simulink model "c28x_xcp_can_3pcaltool"  (R2021b)
settings: Solver=FixedStepDiscrete  StartTime=0.0  StopTime=Inf  RelTol=1e-3  EnableMultiTasking=on
model workspace (MAT data in the model file):
  COUNTER_INCR = Simulink.Parameter
  COUNTER_INCR.Value = 1
  COUNTER_INCR.DataType = 'uint16'
  COUNTER_INCR.Complexity = 'real'
  COUNTER_INCR.Dimensions = [1 1]
  STEP_PARAM = Simulink.Parameter
  STEP_PARAM.Value = 5
  STEP_PARAM.DataType = 'int16'
  STEP_PARAM.Complexity = 'real'
  STEP_PARAM.Dimensions = [1 1]
values from neighbouring files (symbols this model uses):
  STEP_PARAM = tic2000demospkg.Parameter    [c2000_ccp_data.m]
libraries: demo_controls x1
settings Model: ExtModeTrigDuration=8  Creator=The MathWorks, Inc.  LastModifiedBy=The MathWorks, Inc.
settings SolverCC: AlgebraicLoopSolver=TrustRegion  PositivePriorityOrder=on
settings OptimizationCC: DefaultParameterBehavior=Inlined  DefaultUnderspecifiedDataType=single  EnhancedBackFolding=on  PassReuseOutputArgsAs=Individual arguments  MaxStackSize=1024  OptimizeBlockOrder=speed  DifferentSizesBufferReuse=on  OptimizationCustomize=off  DenormalBehavior=FlushToZero  EfficientTunableParamExpr=on
settings DebuggingCC: ParameterTunabilityLossMsg=error  SFMachineParentedDataDiag=warning
settings HardwareCC: ProdBitPerChar=16  ProdBitPerInt=16  ProdBitPerPointer=32  ProdBitPerSizeT=32  ProdBitPerPtrDiffT=32  ProdLargestAtomicInteger=Integer  ProdLargestAtomicFloat=None  ProdWordSize=16  ProdLongLongMode=on  ProdHWDeviceType=Texas Instruments->C2000
settings SFSimCC: MATLABDynamicMemAlloc=off
settings RTWCC: Description=Embedded Coder  SystemTargetFile=ert.tlc  HardwareBoard=TI Delfino F28379D LaunchPad  TemplateMakefile=ert_default_tmf  Toolchain=Texas Instruments Code Composer Studio (C2000)
settings CodeAppCC: ForceParamTrailComments=on  IgnoreCustomStorageClasses=off  OperatorAnnotations=on  SimulinkDataObjDesc=on  SFDataObjDesc=on  InsertBlockDesc=on
settings ERTTargetCC: CodeReplacementLibrary=TI C28x  ExtModeTransport=5  ExtModeStaticAlloc=on  ExtModeStaticAllocSize=10000  ExtModeMexFile=ext_xcp  ExtModeIntrfLevel=Level2 - Open

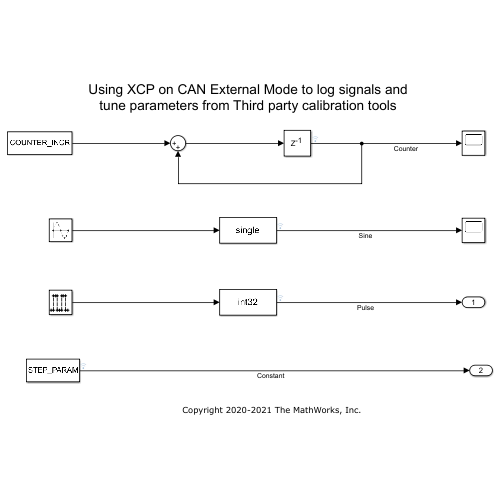
[thumbnail: Simulink's stored preview of the top-level diagram]
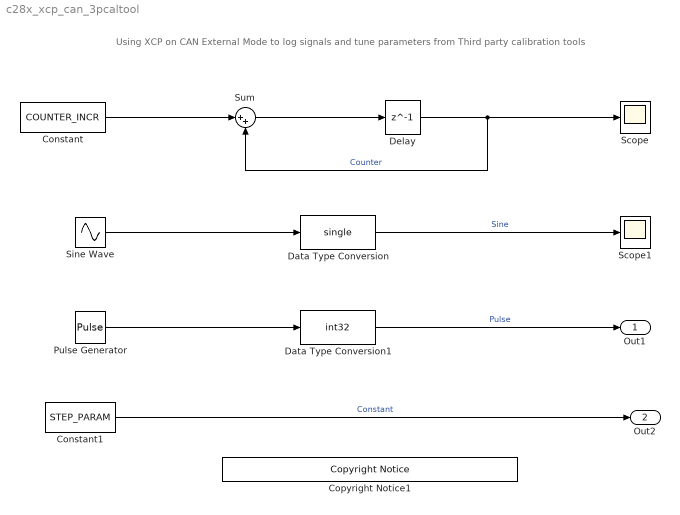
== system c28x_xcp_can_3pcaltool ==
  note: Using XCP on CAN External Mode to log signals and tune parameters from Third party calibration tools
  Constant : Constant  Value=COUNTER_INCR  SampleTime=10e-3
  Constant1 : Constant  Value=STEP_PARAM  SampleTime=10e-3
  Copyright Notice1 : demo_controls/Copyright Notice  year=2020  prod=tic2000
      settings: SourceProductBaseCode=ME
  Data Type Conversion : DataTypeConversion  OutDataTypeStr=single
  Data Type Conversion1 : DataTypeConversion  OutDataTypeStr=int32
  Delay : Delay  DelayLength=1
  Pulse Generator : DiscretePulseGenerator  Amplitude=25  Period=10  PulseWidth=5  SampleTime=50e-3
  Scope : Scope
  Scope1 : Scope
  Sine Wave : Sin  SineType=Sample based  Amplitude=10  Samples=20  SampleTime=10e-3
  Sum : Sum  Inputs=|++
  Out1 : Outport
  Out2 : Outport  Port=2
  wires:
  Delay/1 -> Sum/2, Scope/1  "Counter"
  Sum/1 -> Delay/1
  Constant/1 -> Sum/1
  Sine Wave/1 -> Data Type Conversion/1
  Data Type Conversion/1 -> Scope1/1  "Sine"
  Pulse Generator/1 -> Data Type Conversion1/1
  Data Type Conversion1/1 -> Out1/1  "Pulse"
  Constant1/1 -> Out2/1  "Constant"
